simulink model "SensorFaultInj"  (R2014a)
settings: Solver=FixedStepDiscrete  SolverMode=SingleTasking  StartTime=0.0  StopTime=SimLength  FixedStep=SampleTime  RelTol=1e-3
values from neighbouring files (symbols this model uses):
  GlobalSeed = 10    [set_global_attr.m]
  SampleTime = 0.01    [set_global_attr.m]
  SimLength = 40    [set_global_attr.m]
undefined symbols (not defined in the file or in its folder): actMat, DiscIntNeverNeededParam
libraries: simulink x16, dspswit3 x10
(part 4 of 4)

== system SensorFaultInj/FIM_Muster/Parser Modul/Fault Parameter Parser/Enabled Subsystem/param_fcn id 8/parser_fcn param id 0 ==
  input : Inport
  ex_sfun_paramfcn : S-Function  FunctionName=ex_sfun_paramfcn  EnableBusSupport=off  mask(Legacy Function){SFunctionSpec=double y1 = param_fcn(single u1, single u2, single u3), ShowSpec=on}
      mask prompts: ShowSpec "Display function specification"
      mask help:
      | This block allows you to call the legacy functions specified by the following Legacy Code Tool definition:
      | def.SFunctionName = 'ex_sfun_paramfcn';
      | def.OutputFcnSpec = 'double y1 = param_fcn(single u1, single u2, single u3)';
      | def.HeaderFiles = {'param_fcn.hpp'};
      | def.SourceFiles = {'param_fcn.cpp'};
      | def.Options.language = 'C++';
      mask Help: <p>This block was generated automatically by the Legacy Code Tool. For detailed help on this tool, call<a href="matlab:legacy_code('help')"> legacy_code('help')</a>.</p>
      mask Callback ShowSpec:
      | if strcmp(get_param(gcbh, 'ShowSpec'), 'on')
      |   set_param(gcbh, 'MaskDisplay', sprintf('fprintf(''%s'');', get_param(gcbh, 'SFunctionSpec')));
      | else
      |   set_param(gcbh, 'MaskDisplay', sprintf('fprintf(''%s'');', get_param(gcbh, 'FunctionName')));
      | end
      mask Display: fprintf('double y1 = param_fcn(single u1, single u2, single u3)');
  "fault_id " : Constant  Value=8  OutDataTypeStr=single
  "param_id " : Constant  Value=0  OutDataTypeStr=single
  output : Outport
  wires:
  "fault_id "/1 -> ex_sfun_paramfcn/1
  "param_id "/1 -> ex_sfun_paramfcn/2
  ex_sfun_paramfcn/1 -> output/1
  input/1 -> ex_sfun_paramfcn/3

== system SensorFaultInj/FIM_Muster/Parser Modul/Fault Parameter Parser/Enabled Subsystem/param_fcn id 9/parser_fcn param id 1 ==
  input : Inport
  ex_sfun_paramfcn : S-Function  FunctionName=ex_sfun_paramfcn  EnableBusSupport=off  mask(Legacy Function){SFunctionSpec=double y1 = param_fcn(single u1, single u2, single u3), ShowSpec=on}
      mask prompts: ShowSpec "Display function specification"
      mask help:
      | This block allows you to call the legacy functions specified by the following Legacy Code Tool definition:
      | def.SFunctionName = 'ex_sfun_paramfcn';
      | def.OutputFcnSpec = 'double y1 = param_fcn(single u1, single u2, single u3)';
      | def.HeaderFiles = {'param_fcn.hpp'};
      | def.SourceFiles = {'param_fcn.cpp'};
      | def.Options.language = 'C++';
      mask Help: <p>This block was generated automatically by the Legacy Code Tool. For detailed help on this tool, call<a href="matlab:legacy_code('help')"> legacy_code('help')</a>.</p>
      mask Callback ShowSpec:
      | if strcmp(get_param(gcbh, 'ShowSpec'), 'on')
      |   set_param(gcbh, 'MaskDisplay', sprintf('fprintf(''%s'');', get_param(gcbh, 'SFunctionSpec')));
      | else
      |   set_param(gcbh, 'MaskDisplay', sprintf('fprintf(''%s'');', get_param(gcbh, 'FunctionName')));
      | end
      mask Display: fprintf('double y1 = param_fcn(single u1, single u2, single u3)');
  "fault_id " : Constant  Value=9  OutDataTypeStr=single
  "param_id " : Constant  Value=2  OutDataTypeStr=single
  output : Outport
  wires:
  "fault_id "/1 -> ex_sfun_paramfcn/1
  "param_id "/1 -> ex_sfun_paramfcn/2
  ex_sfun_paramfcn/1 -> output/1
  input/1 -> ex_sfun_paramfcn/3

== system SensorFaultInj/FIM_Muster/Parser Modul/Fault Parameter Parser/Enabled Subsystem/param_fcn id 9/parser_fcn param id 2 ==
  input : Inport
  ex_sfun_paramfcn : S-Function  FunctionName=ex_sfun_paramfcn  EnableBusSupport=off  mask(Legacy Function){SFunctionSpec=double y1 = param_fcn(single u1, single u2, single u3), ShowSpec=on}
      mask prompts: ShowSpec "Display function specification"
      mask help:
      | This block allows you to call the legacy functions specified by the following Legacy Code Tool definition:
      | def.SFunctionName = 'ex_sfun_paramfcn';
      | def.OutputFcnSpec = 'double y1 = param_fcn(single u1, single u2, single u3)';
      | def.HeaderFiles = {'param_fcn.hpp'};
      | def.SourceFiles = {'param_fcn.cpp'};
      | def.Options.language = 'C++';
      mask Help: <p>This block was generated automatically by the Legacy Code Tool. For detailed help on this tool, call<a href="matlab:legacy_code('help')"> legacy_code('help')</a>.</p>
      mask Callback ShowSpec:
      | if strcmp(get_param(gcbh, 'ShowSpec'), 'on')
      |   set_param(gcbh, 'MaskDisplay', sprintf('fprintf(''%s'');', get_param(gcbh, 'SFunctionSpec')));
      | else
      |   set_param(gcbh, 'MaskDisplay', sprintf('fprintf(''%s'');', get_param(gcbh, 'FunctionName')));
      | end
      mask Display: fprintf('double y1 = param_fcn(single u1, single u2, single u3)');
  "fault_id " : Constant  Value=9  OutDataTypeStr=single
  "param_id " : Constant  Value=0  OutDataTypeStr=single
  output : Outport
  wires:
  "fault_id "/1 -> ex_sfun_paramfcn/1
  "param_id "/1 -> ex_sfun_paramfcn/2
  ex_sfun_paramfcn/1 -> output/1
  input/1 -> ex_sfun_paramfcn/3

== system SensorFaultInj/FIM_Muster/Parser Modul/Fault Parameter Parser/Enabled Subsystem/param_fcn id 9/parser_fcn param id 3 ==
  input : Inport
  ex_sfun_paramfcn : S-Function  FunctionName=ex_sfun_paramfcn  EnableBusSupport=off  mask(Legacy Function){SFunctionSpec=double y1 = param_fcn(single u1, single u2, single u3), ShowSpec=on}
      mask prompts: ShowSpec "Display function specification"
      mask help:
      | This block allows you to call the legacy functions specified by the following Legacy Code Tool definition:
      | def.SFunctionName = 'ex_sfun_paramfcn';
      | def.OutputFcnSpec = 'double y1 = param_fcn(single u1, single u2, single u3)';
      | def.HeaderFiles = {'param_fcn.hpp'};
      | def.SourceFiles = {'param_fcn.cpp'};
      | def.Options.language = 'C++';
      mask Help: <p>This block was generated automatically by the Legacy Code Tool. For detailed help on this tool, call<a href="matlab:legacy_code('help')"> legacy_code('help')</a>.</p>
      mask Callback ShowSpec:
      | if strcmp(get_param(gcbh, 'ShowSpec'), 'on')
      |   set_param(gcbh, 'MaskDisplay', sprintf('fprintf(''%s'');', get_param(gcbh, 'SFunctionSpec')));
      | else
      |   set_param(gcbh, 'MaskDisplay', sprintf('fprintf(''%s'');', get_param(gcbh, 'FunctionName')));
      | end
      mask Display: fprintf('double y1 = param_fcn(single u1, single u2, single u3)');
  "fault_id " : Constant  Value=9  OutDataTypeStr=single
  "param_id " : Constant  OutDataTypeStr=single
  output : Outport
  wires:
  "fault_id "/1 -> ex_sfun_paramfcn/1
  "param_id "/1 -> ex_sfun_paramfcn/2
  ex_sfun_paramfcn/1 -> output/1
  input/1 -> ex_sfun_paramfcn/3
